simulink model "exLongLinePV_sim"  (R2014b)
settings: Solver=ode45  SolverMode=SingleTasking  StartTime=0.0  StopTime=1.5  MaxStep=0.0015  RelTol=0.0001
values from neighbouring files (symbols this model uses):
  At = full(At)    [exLongLinePV.m]
  Bt = full(Bt)    [exLongLinePV.m]
  bus1_vd = 2^0.5*1e3    (= 1414.21356237)    [ex3busPV.m]    (also in exLongLinePV.m = 141421.356237)
  bus1_vq = 0    [ex3busPV.m]    (also in exLongLinePV.m)
  Cbus = [600e-6 ; 600e-6]    [ex14busSGandPV.m]    (also in exLongLinePV.m = 0.001)
  Cgen = 2e-3*Pren/(gen_vd_init^2+gen_vq_init^2)    (= 5e-07)    [ex3busPV.m]    (also in exLongLinePV.m = 2e-07)
  Ct = full(Ct)    [exLongLinePV.m]
  Dt = full(Dt)    [exLongLinePV.m]
  ki = [0.3 ; 0.3]    [ex14busSGandPV.m]    (also in exLongLinePV.m = 1e-05)
  kp = [1.3e-6 ; 1.3e-6]    [ex14busSGandPV.m]    (also in exLongLinePV.m = 1e-05)
  Pren = [10 ; 10]*1e6    [ex14busSGandPV.m]    (also in ex3busPV.m = 500; exLongLinePV.m = 5000000)
  rel_step = 0.6    [ex3busPV.m]    (also in exLongLinePV.m = 0.02; syncMachVsSwing.m = 1)
  step_time = 9    [ex2busStability.m]    (also in ex3busPV.m = 0.05; exDroopB.m = 10; exLongLinePV.m = 1; syncMachVsSwing.m = 5)
  Vbus_ref = [800 ; 800]    [ex14busSGandPV.m]    (also in exLongLinePV.m = 800)
  ws = 2*pi*50    (= 314.159265359)    [ex14busSGandPV.m]    (also in ex2busStability.m; ex3busPV.m; ex7busLongLine.m; ex9busSG.m)
libraries: simulink x1
settings Model: Creator=COPEC  LastModifiedBy=Juri
settings OptimizationCC: BlockReduction=off  BooleanDataType=off
settings DebuggingCC: SaveWithParameterizedLinksMsg=none  UnderspecifiedInitializationDetection=Classic  MergeDetectMultiDrivingBlocksExec=none  SignalResolutionControl=TryResolveAllWithWarning  SolverPrmCheckMsg=none  FrameProcessingCompatibilityMsg=error
settings HardwareCC: TargetUnknown=on

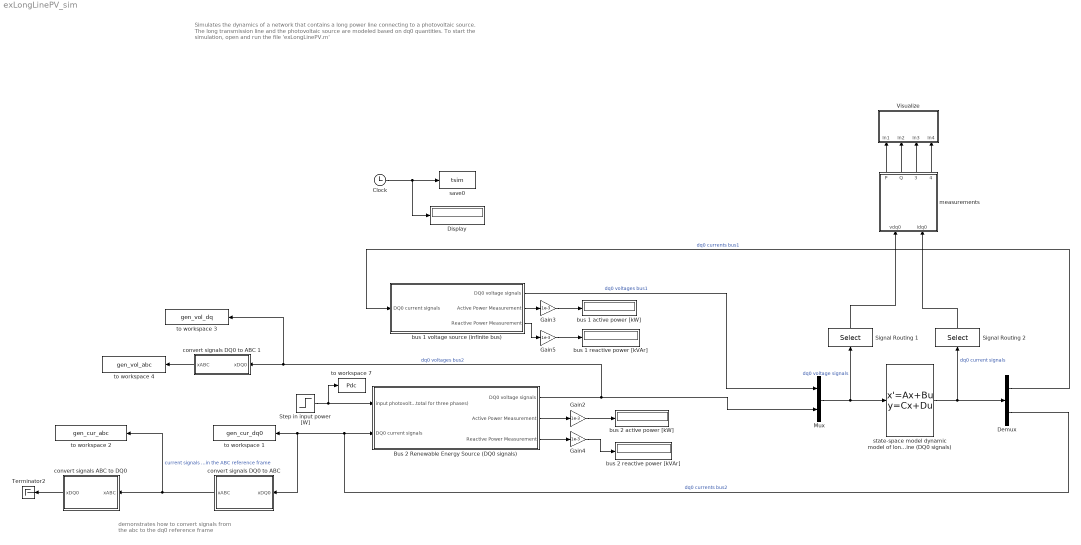
== system exLongLinePV_sim ==
  note: demonstrates how to convert signals
      | from the abc to the dq0 reference frame
  note: Simulates the dynamics of a network that contains
      | a long power line connecting to a photovoltaic source.
      | The long transmission line and the photovoltaic source are modeled
      | based on dq0 quantities.
      |
      | To start the simulation, open and run the file
      | 'exLongLinePV.m'
  Bus 2 Renewable Energy Source (DQ0 signals) : Subsystem
  Clock : Clock
  Demux : Demux  Outputs=2
  Display : Display
  Gain{2..5} (4 alike) : Gain  Gain=1e-3
  Mux : Mux  Inputs=2
  "Signal Routing 1 " : Selector  InputPortWidth=6  IndexOptions=Index vector (dialog)  Indices=[1 4 2 5 3 6]  OutputSizes=1
  Signal Routing 2 : Selector  InputPortWidth=6  IndexOptions=Index vector (dialog)  Indices=[1 4 2 5 3 6]  OutputSizes=1
  Step in input power [W] : Step  Time=step_time  Before=3*Pren  After=3*Pren*(1+rel_step)  SampleTime=0
  Terminator2 : Terminator
  Visualize : Subsystem
  bus 1 voltage source (infinite bus) : Subsystem
  bus 1 active power [kW] : Display
  bus 1 reactive power [kVAr] : Display
  bus 2 active power [kW] : Display
  bus 2 reactive power [kVAr] : Display
  convert signals ABC to DQ0 : Subsystem
  convert signals DQ0 to ABC : Subsystem
  convert signals DQ0 to ABC 1 : Subsystem
  measurements : Subsystem
  save0 : ToWorkspace  VariableName=tsim  SampleTime=-1
  state-space model dynamic model of long transmission line (DQ0 signals) : StateSpace  A=At  B=Bt  C=Ct  D=Dt  X0=0
  to workspace 1 : ToWorkspace  VariableName=gen_cur_dq0  SampleTime=-1
  to workspace 2 : ToWorkspace  VariableName=gen_cur_abc  SampleTime=-1
  to workspace 3 : ToWorkspace  VariableName=gen_vol_dq  SampleTime=-1
  to workspace 4 : ToWorkspace  VariableName=gen_vol_abc  SampleTime=-1
  to workspace 7 : ToWorkspace  VariableName=Pdc  SampleTime=-1
  wires:
  Clock/1 -> Display/1, save0/1
  Gain2/1 -> bus 2 active power [kW]/1
  Gain4/1 -> bus 2 reactive power [kVAr]/1
  Step in input power [W]/1 -> to workspace 7/1, Bus 2 Renewable Energy Source (DQ0 signals)/1(input photovoltaic power (total for three phases))
  Bus 2 Renewable Energy Source (DQ0 signals)/2(Active Power Measurement) -> Gain2/1
  Bus 2 Renewable Energy Source (DQ0 signals)/3("Reactive Power Measurement ") -> Gain4/1
  Mux/1 -> state-space model dynamic model of long transmission line (DQ0 signals)/1, "Signal Routing 1 "/1  "dq0 voltage signals"
  bus 1 voltage source (infinite bus)/1(DQ0 voltage signals) -> Mux/1  "dq0 voltages bus1"
  Bus 2 Renewable Energy Source (DQ0 signals)/1(DQ0 voltage signals) -> to workspace 3/1, convert signals DQ0 to ABC 1/1(xDQ0), Mux/2  "dq0 voltages bus2"
  Demux/1 -> bus 1 voltage source (infinite bus)/1(DQ0 current signals)  "dq0 currents bus1"
  Demux/2 -> Bus 2 Renewable Energy Source (DQ0 signals)/2(DQ0 current signals), convert signals DQ0 to ABC/1(xDQ0), to workspace 1/1  "dq0 currents bus2"
  state-space model dynamic model of long transmission line (DQ0 signals)/1 -> Demux/1, Signal Routing 2/1  "dq0 current signals"
  convert signals DQ0 to ABC/1(xABC) -> to workspace 2/1, convert signals ABC to DQ0/1(xABC)  "current signals in the ABC reference frame"
  convert signals ABC to DQ0/1(xDQ0) -> Terminator2/1
  convert signals DQ0 to ABC 1/1(xABC) -> to workspace 4/1
  bus 1 voltage source (infinite bus)/2(Active Power Measurement) -> Gain3/1
  bus 1 voltage source (infinite bus)/3("Reactive Power Measurement ") -> Gain5/1
  Gain3/1 -> bus 1 active power [kW]/1
  Gain5/1 -> bus 1 reactive power [kVAr]/1
  "Signal Routing 1 "/1 -> measurements/1(vdq0)
  Signal Routing 2/1 -> measurements/2(idq0)
  measurements/1(P) -> Visualize/1(In1)
  measurements/2(Q) -> Visualize/2(In2)
  measurements/3(Vm_RMS) -> Visualize/3(In3)
  measurements/4(Vph_deg) -> Visualize/4(In4)

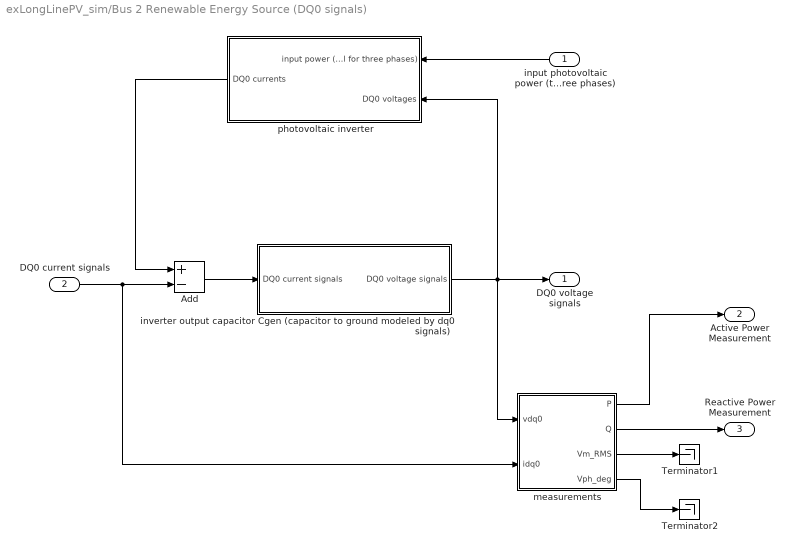
== system exLongLinePV_sim/Bus 2 Renewable Energy Source (DQ0 signals) ==
  input photovoltaic power (total for three phases) : Inport
  DQ0 current signals : Inport  Port=2
  Add : Sum  Inputs=+-
  Terminator1 : Terminator
  Terminator2 : Terminator
  inverter output capacitor Cgen (capacitor to ground modeled by dq0 signals) : Subsystem
  measurements : Subsystem
  photovoltaic inverter : Subsystem
  DQ0 voltage signals : Outport
  Active Power Measurement : Outport  Port=2
  "Reactive Power Measurement " : Outport  Port=3
  wires:
  DQ0 current signals/1 -> Add/2, measurements/2(idq0)
  inverter output capacitor Cgen (capacitor to ground modeled by dq0 signals)/1(DQ0 voltage signals) -> photovoltaic inverter/2(DQ0 voltages), DQ0 voltage signals/1, measurements/1(vdq0)
  input photovoltaic power (total for three phases)/1 -> photovoltaic inverter/1(input power (total for three phases))
  photovoltaic inverter/1(DQ0 currents) -> Add/1
  Add/1 -> inverter output capacitor Cgen (capacitor to ground modeled by dq0 signals)/1(DQ0 current signals)
  measurements/1(P) -> Active Power Measurement/1
  measurements/2(Q) -> "Reactive Power Measurement "/1
  measurements/3(Vm_RMS) -> Terminator1/1
  measurements/4(Vph_deg) -> Terminator2/1

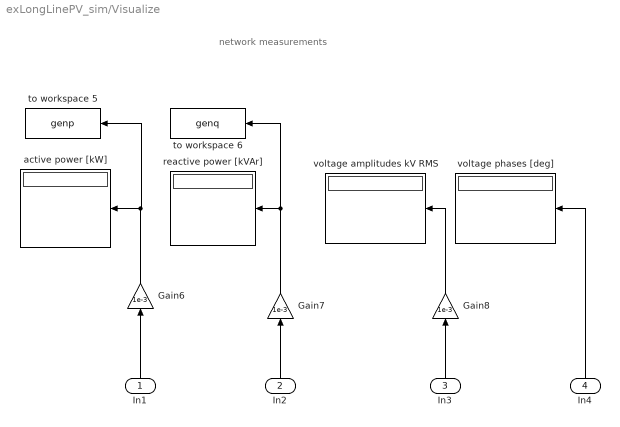
== system exLongLinePV_sim/Visualize ==
  note: network measurements
  In1 : Inport
  In2 : Inport  Port=2
  In3 : Inport  Port=3
  In4 : Inport  Port=4
  Gain6 : Gain  Gain=1e-3
  Gain7 : Gain  Gain=1e-3
  Gain8 : Gain  Gain=1e-3
  active power [kW] : Display
  reactive power [kVAr] : Display
  to workspace 5 : ToWorkspace  VariableName=genp  SampleTime=-1
  to workspace 6 : ToWorkspace  VariableName=genq  SampleTime=-1
  "voltage amplitudes kV RMS " : Display
  voltage phases [deg] : Display
  wires:
  In2/1 -> Gain7/1
  In3/1 -> Gain8/1
  Gain7/1 -> to workspace 6/1, reactive power [kVAr]/1
  In1/1 -> Gain6/1
  Gain8/1 -> "voltage amplitudes kV RMS "/1
  Gain6/1 -> to workspace 5/1, active power [kW]/1
  In4/1 -> voltage phases [deg]/1

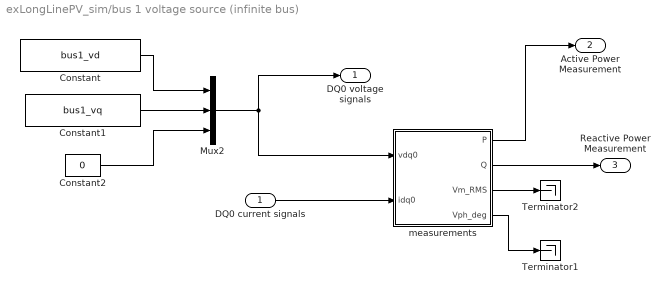
== system exLongLinePV_sim/bus 1 voltage source (infinite bus) ==
  DQ0 current signals : Inport
  Constant : Constant  Value=bus1_vd
  Constant1 : Constant  Value=bus1_vq
  Constant2 : Constant  Value=0
  Mux2 : Mux  Inputs=3
  Terminator1 : Terminator
  Terminator2 : Terminator
  measurements : Subsystem
  DQ0 voltage signals : Outport
  Active Power Measurement : Outport  Port=2
  "Reactive Power Measurement " : Outport  Port=3
  wires:
  Constant/1 -> Mux2/1
  Constant1/1 -> Mux2/2
  Constant2/1 -> Mux2/3
  Mux2/1 -> measurements/1(vdq0), DQ0 voltage signals/1
  DQ0 current signals/1 -> measurements/2(idq0)
  measurements/1(P) -> Active Power Measurement/1
  measurements/2(Q) -> "Reactive Power Measurement "/1
  measurements/3(Vm_RMS) -> Terminator2/1
  measurements/4(Vph_deg) -> Terminator1/1

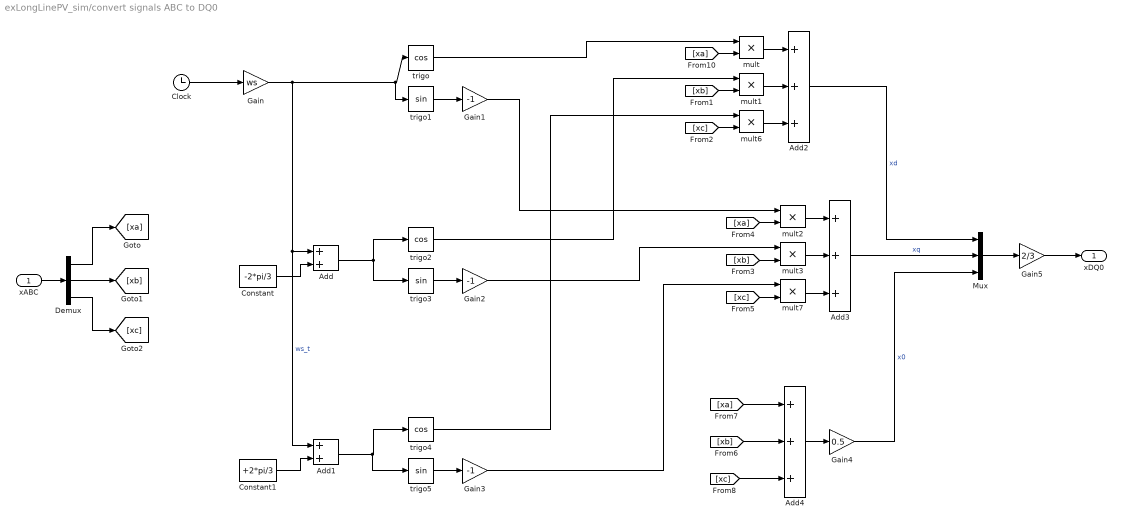
== system exLongLinePV_sim/convert signals ABC to DQ0 ==
  xABC : Inport
  Add : Sum
  Add1 : Sum
  Add2 : Sum  Inputs=+++
  Add3 : Sum  Inputs=+++
  Add4 : Sum  Inputs=+++
  Clock : Clock
  Constant : Constant  Value=-2*pi/3
  Constant1 : Constant  Value=+2*pi/3
  Demux : Demux  Outputs=3
  Gain : Gain  Gain=ws
  Gain1 : Gain  Gain=-1
  Gain2 : Gain  Gain=-1
  Gain3 : Gain  Gain=-1
  Gain4 : Gain  Gain=0.5
  Gain5 : Gain  Gain=2/3
  Mux : Mux  Inputs=3
  mult{,1..3,6..7} (6 alike) : Product  Inputs=**
  trigo : Trigonometry  Operator=cos
  trigo1 : Trigonometry
  trigo2 : Trigonometry  Operator=cos
  trigo3 : Trigonometry
  trigo4 : Trigonometry  Operator=cos
  trigo5 : Trigonometry
  xDQ0 : Outport
  wires:
  Gain5/1 -> xDQ0/1
  Mux/1 -> Gain5/1
  Gain3/1 -> mult7/1
  Gain2/1 -> mult3/1
  Gain1/1 -> mult2/1
  [xc] -> Add4/3
  [xb] -> Add4/2
  [xa] -> Add4/1
  Add4/1 -> Gain4/1
  mult7/1 -> Add3/3
  [xc] -> mult7/2
  [xb] -> mult3/2
  [xa] -> mult2/2
  trigo4/1 -> mult6/1
  mult6/1 -> Add2/3
  [xc] -> mult6/2
  trigo2/1 -> mult1/1
  trigo/1 -> mult/1
  Gain4/1 -> Mux/3  "x0"
  Add3/1 -> Mux/2  "xq"
  Add2/1 -> Mux/1  "xd"
  mult3/1 -> Add3/2
  mult2/1 -> Add3/1
  [xb] -> mult1/2
  [xa] -> mult/2
  mult1/1 -> Add2/2
  mult/1 -> Add2/1
  Demux/3 -> [xc]
  Demux/2 -> [xb]
  Demux/1 -> [xa]
  xABC/1 -> Demux/1
  Add1/1 -> trigo4/1, trigo5/1
  trigo5/1 -> Gain3/1
  Add/1 -> trigo3/1, trigo2/1
  trigo3/1 -> Gain2/1
  trigo1/1 -> Gain1/1
  Constant1/1 -> Add1/2
  Constant/1 -> Add/2
  Gain/1 -> Add/1, Add1/1, trigo/1, trigo1/1  "ws_t"
  Clock/1 -> Gain/1

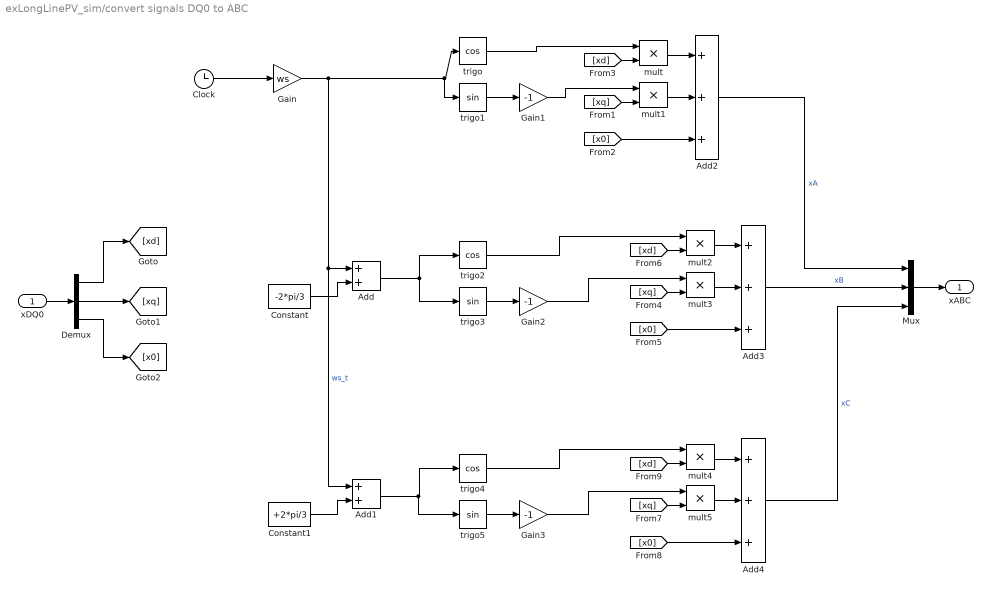
== system exLongLinePV_sim/convert signals DQ0 to ABC ==
  xDQ0 : Inport
  Add : Sum
  Add1 : Sum
  Add2 : Sum  Inputs=+++
  Add3 : Sum  Inputs=+++
  Add4 : Sum  Inputs=+++
  Clock : Clock
  Constant : Constant  Value=-2*pi/3
  Constant1 : Constant  Value=+2*pi/3
  Demux : Demux  Outputs=3
  Gain : Gain  Gain=ws
  Gain1 : Gain  Gain=-1
  Gain2 : Gain  Gain=-1
  Gain3 : Gain  Gain=-1
  Mux : Mux  Inputs=3
  mult{,1..5} (6 alike) : Product  Inputs=**
  trigo : Trigonometry  Operator=cos
  trigo1 : Trigonometry
  trigo2 : Trigonometry  Operator=cos
  trigo3 : Trigonometry
  trigo4 : Trigonometry  Operator=cos
  trigo5 : Trigonometry
  xABC : Outport
  wires:
  Clock/1 -> Gain/1
  Gain/1 -> trigo1/1, trigo/1, Add1/1, Add/1  "ws_t"
  Constant/1 -> Add/2
  Constant1/1 -> Add1/2
  trigo1/1 -> Gain1/1
  trigo3/1 -> Gain2/1
  Add/1 -> trigo2/1, trigo3/1
  trigo5/1 -> Gain3/1
  Add1/1 -> trigo5/1, trigo4/1
  xDQ0/1 -> Demux/1
  Demux/1 -> [xd]
  Demux/2 -> [xq]
  Demux/3 -> [x0]
  Mux/1 -> xABC/1
  mult/1 -> Add2/1
  mult1/1 -> Add2/2
  [xd] -> mult/2
  [xq] -> mult1/2
  [x0] -> Add2/3
  mult2/1 -> Add3/1
  mult3/1 -> Add3/2
  [xd] -> mult2/2
  [xq] -> mult3/2
  [x0] -> Add3/3
  mult4/1 -> Add4/1
  mult5/1 -> Add4/2
  [xd] -> mult4/2
  [xq] -> mult5/2
  [x0] -> Add4/3
  trigo/1 -> mult/1
  Gain1/1 -> mult1/1
  trigo2/1 -> mult2/1
  Gain2/1 -> mult3/1
  trigo4/1 -> mult4/1
  Gain3/1 -> mult5/1
  Add2/1 -> Mux/1  "xA"
  Add3/1 -> Mux/2  "xB"
  Add4/1 -> Mux/3  "xC"

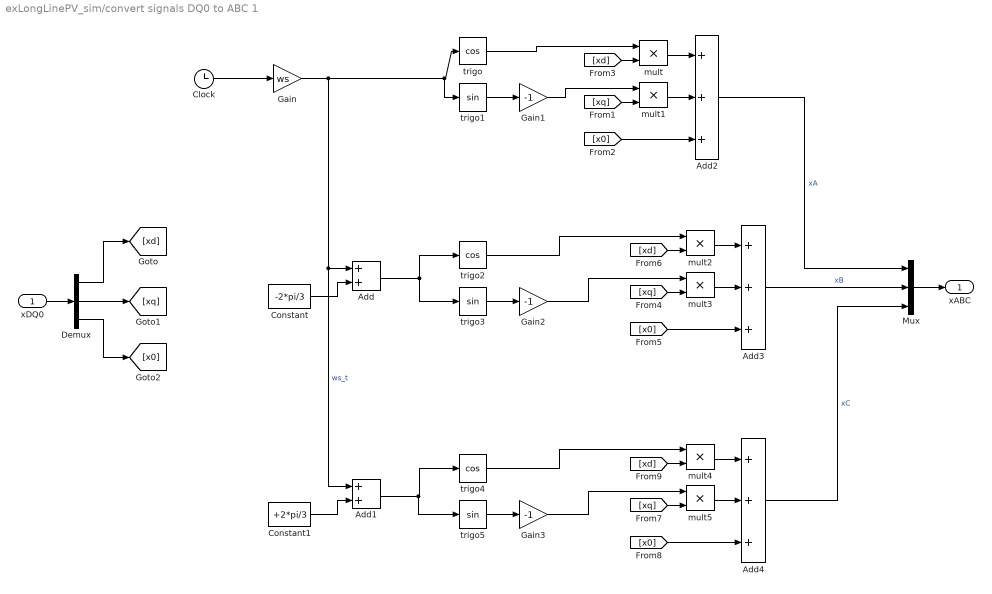
== system exLongLinePV_sim/convert signals DQ0 to ABC 1 ==
  xDQ0 : Inport
  Add : Sum
  Add1 : Sum
  Add2 : Sum  Inputs=+++
  Add3 : Sum  Inputs=+++
  Add4 : Sum  Inputs=+++
  Clock : Clock
  Constant : Constant  Value=-2*pi/3
  Constant1 : Constant  Value=+2*pi/3
  Demux : Demux  Outputs=3
  Gain : Gain  Gain=ws
  Gain1 : Gain  Gain=-1
  Gain2 : Gain  Gain=-1
  Gain3 : Gain  Gain=-1
  Mux : Mux  Inputs=3
  mult{,1..5} (6 alike) : Product  Inputs=**
  trigo : Trigonometry  Operator=cos
  trigo1 : Trigonometry
  trigo2 : Trigonometry  Operator=cos
  trigo3 : Trigonometry
  trigo4 : Trigonometry  Operator=cos
  trigo5 : Trigonometry
  xABC : Outport
  wires:
  Clock/1 -> Gain/1
  Gain/1 -> trigo1/1, trigo/1, Add1/1, Add/1  "ws_t"
  Constant/1 -> Add/2
  Constant1/1 -> Add1/2
  trigo1/1 -> Gain1/1
  trigo3/1 -> Gain2/1
  Add/1 -> trigo2/1, trigo3/1
  trigo5/1 -> Gain3/1
  Add1/1 -> trigo5/1, trigo4/1
  xDQ0/1 -> Demux/1
  Demux/1 -> [xd]
  Demux/2 -> [xq]
  Demux/3 -> [x0]
  Mux/1 -> xABC/1
  mult/1 -> Add2/1
  mult1/1 -> Add2/2
  [xd] -> mult/2
  [xq] -> mult1/2
  [x0] -> Add2/3
  mult2/1 -> Add3/1
  mult3/1 -> Add3/2
  [xd] -> mult2/2
  [xq] -> mult3/2
  [x0] -> Add3/3
  mult4/1 -> Add4/1
  mult5/1 -> Add4/2
  [xd] -> mult4/2
  [xq] -> mult5/2
  [x0] -> Add4/3
  trigo/1 -> mult/1
  Gain1/1 -> mult1/1
  trigo2/1 -> mult2/1
  Gain2/1 -> mult3/1
  trigo4/1 -> mult4/1
  Gain3/1 -> mult5/1
  Add2/1 -> Mux/1  "xA"
  Add3/1 -> Mux/2  "xB"
  Add4/1 -> Mux/3  "xC"

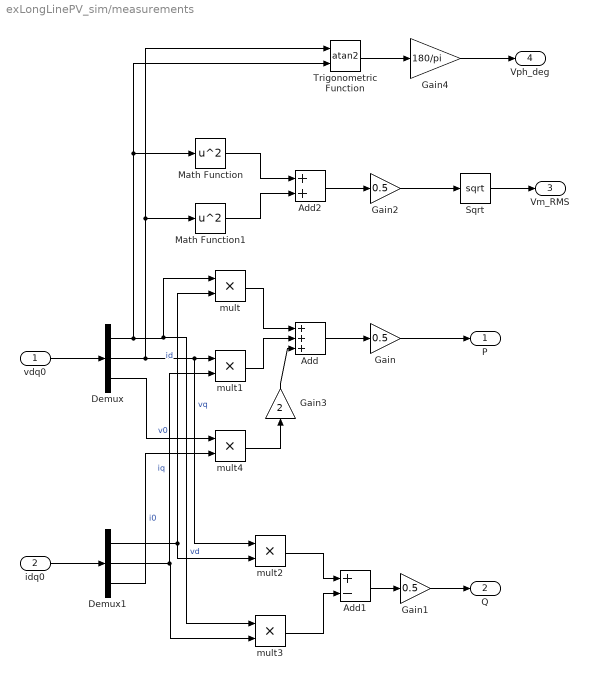
== system exLongLinePV_sim/measurements ==
  vdq0 : Inport
  idq0 : Inport  Port=2
  Add : Sum  Inputs=+++
  Add1 : Sum  Inputs=+-
  Add2 : Sum
  Demux : Demux  Outputs=3
  Demux1 : Demux  Outputs=3
  Gain : Gain  Gain=0.5
  Gain1 : Gain  Gain=0.5
  Gain2 : Gain  Gain=0.5
  Gain3 : Gain  Gain=2
  Gain4 : Gain  Gain=180/pi
  Math Function : Math  Operator=square  SaturateOnIntegerOverflow=on
  Math Function1 : Math  Operator=square  SaturateOnIntegerOverflow=on
  Sqrt : Sqrt  SaturateOnIntegerOverflow=on
  Trigonometric Function : Trigonometry  Operator=atan2
  mult{,1..4} (5 alike) : Product  Inputs=**
  P : Outport
  Q : Outport  Port=2
  Vm_RMS : Outport  Port=3
  Vph_deg : Outport  Port=4
  wires:
  idq0/1 -> Demux1/1
  vdq0/1 -> Demux/1
  Demux/1 -> Math Function/1, Trigonometric Function/2, mult3/1, mult/1  "vd"
  Demux/2 -> Trigonometric Function/1, Math Function1/1, mult2/1, mult1/1  "vq"
  Demux1/1 -> mult/2, mult2/2  "id"
  Demux1/2 -> mult3/2, mult1/2  "iq"
  Demux/3 -> mult4/1  "v0"
  Demux1/3 -> mult4/2  "i0"
  mult/1 -> Add/1
  mult1/1 -> Add/2
  Add/1 -> Gain/1
  mult2/1 -> Add1/1
  mult3/1 -> Add1/2
  Add1/1 -> Gain1/1
  Sqrt/1 -> Vm_RMS/1
  Math Function/1 -> Add2/1
  Math Function1/1 -> Add2/2
  Add2/1 -> Gain2/1
  Gain2/1 -> Sqrt/1
  Gain/1 -> P/1
  Gain1/1 -> Q/1
  mult4/1 -> Gain3/1
  Gain3/1 -> Add/3
  Trigonometric Function/1 -> Gain4/1
  Gain4/1 -> Vph_deg/1

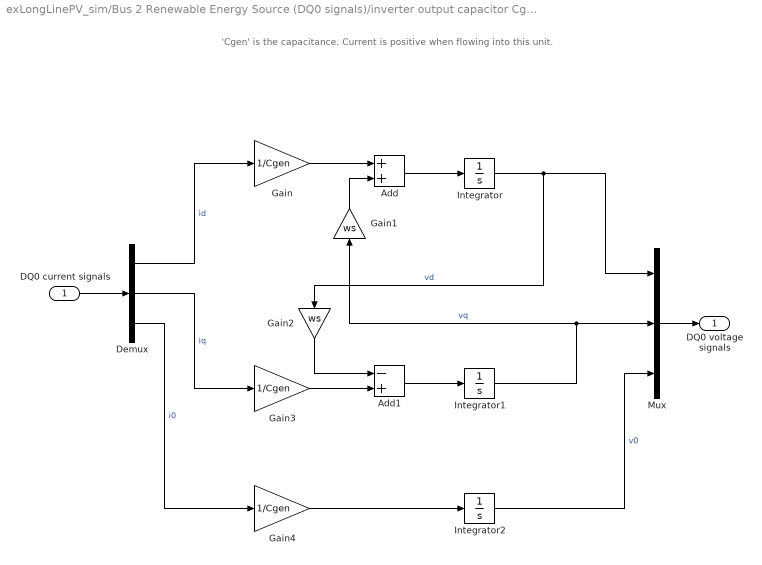
== system exLongLinePV_sim/Bus 2 Renewable Energy Source (DQ0 signals)/inverter output capacitor Cgen (capacitor to ground modeled by dq0 signals) ==
  note: 'Cgen' is the capacitance.
      | Current is positive when flowing into this unit.
  DQ0 current signals : Inport
  Add : Sum
  Add1 : Sum  Inputs=-+
  Demux : Demux  Outputs=3
  Gain : Gain  Gain=1/Cgen
  Gain1 : Gain  Gain=ws
  Gain2 : Gain  Gain=ws
  Gain3 : Gain  Gain=1/Cgen
  Gain4 : Gain  Gain=1/Cgen
  Integrator : Integrator  InitialCondition=bus1_vd
  Integrator1 : Integrator  InitialCondition=bus1_vq
  Integrator2 : Integrator
  Mux : Mux  Inputs=3
  DQ0 voltage signals : Outport
  wires:
  Integrator2/1 -> Mux/3  "v0"
  Mux/1 -> DQ0 voltage signals/1
  Integrator/1 -> Gain2/1, Mux/1  "vd"
  Integrator1/1 -> Gain1/1, Mux/2  "vq"
  Add/1 -> Integrator/1
  Gain1/1 -> Add/2
  DQ0 current signals/1 -> Demux/1
  Demux/1 -> Gain/1  "id"
  Gain/1 -> Add/1
  Add1/1 -> Integrator1/1
  Gain2/1 -> Add1/1
  Demux/2 -> Gain3/1  "iq"
  Gain3/1 -> Add1/2
  Demux/3 -> Gain4/1  "i0"
  Gain4/1 -> Integrator2/1

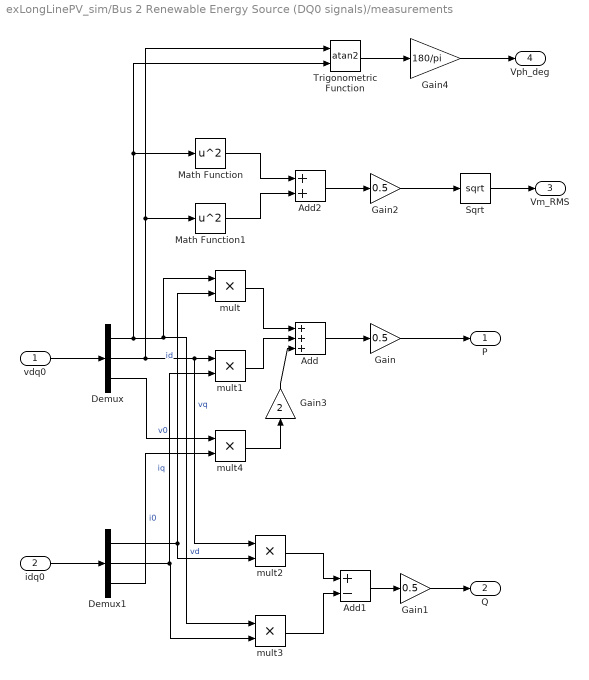
== system exLongLinePV_sim/Bus 2 Renewable Energy Source (DQ0 signals)/measurements ==
  vdq0 : Inport
  idq0 : Inport  Port=2
  Add : Sum  Inputs=+++
  Add1 : Sum  Inputs=+-
  Add2 : Sum
  Demux : Demux  Outputs=3
  Demux1 : Demux  Outputs=3
  Gain : Gain  Gain=0.5
  Gain1 : Gain  Gain=0.5
  Gain2 : Gain  Gain=0.5
  Gain3 : Gain  Gain=2
  Gain4 : Gain  Gain=180/pi
  Math Function : Math  Operator=square  SaturateOnIntegerOverflow=on
  Math Function1 : Math  Operator=square  SaturateOnIntegerOverflow=on
  Sqrt : Sqrt  SaturateOnIntegerOverflow=on
  Trigonometric Function : Trigonometry  Operator=atan2
  mult{,1..4} (5 alike) : Product  Inputs=**
  P : Outport
  Q : Outport  Port=2
  Vm_RMS : Outport  Port=3
  Vph_deg : Outport  Port=4
  wires:
  idq0/1 -> Demux1/1
  vdq0/1 -> Demux/1
  Demux/1 -> Math Function/1, Trigonometric Function/2, mult3/1, mult/1  "vd"
  Demux/2 -> Trigonometric Function/1, Math Function1/1, mult2/1, mult1/1  "vq"
  Demux1/1 -> mult/2, mult2/2  "id"
  Demux1/2 -> mult3/2, mult1/2  "iq"
  Demux/3 -> mult4/1  "v0"
  Demux1/3 -> mult4/2  "i0"
  mult/1 -> Add/1
  mult1/1 -> Add/2
  Add/1 -> Gain/1
  mult2/1 -> Add1/1
  mult3/1 -> Add1/2
  Add1/1 -> Gain1/1
  Sqrt/1 -> Vm_RMS/1
  Math Function/1 -> Add2/1
  Math Function1/1 -> Add2/2
  Add2/1 -> Gain2/1
  Gain2/1 -> Sqrt/1
  Gain/1 -> P/1
  Gain1/1 -> Q/1
  mult4/1 -> Gain3/1
  Gain3/1 -> Add/3
  Trigonometric Function/1 -> Gain4/1
  Gain4/1 -> Vph_deg/1

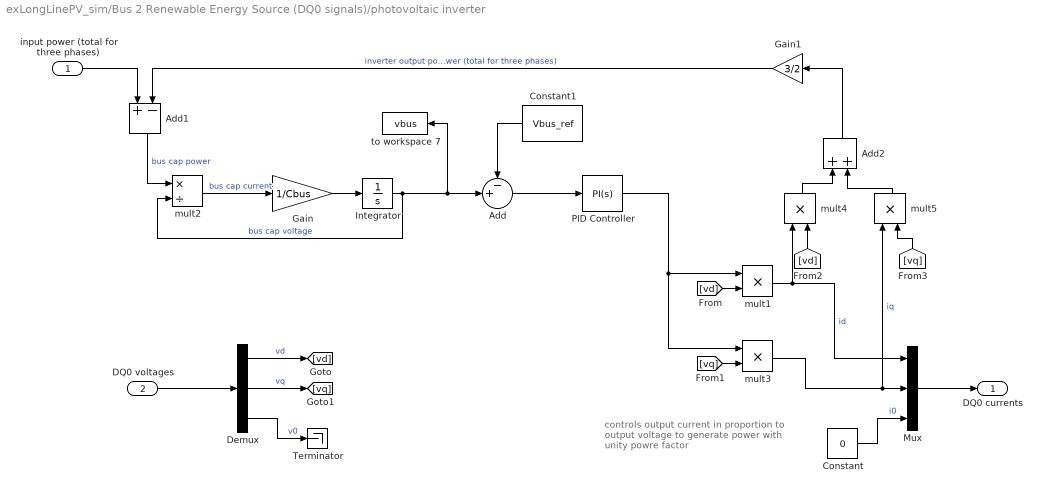
== system exLongLinePV_sim/Bus 2 Renewable Energy Source (DQ0 signals)/photovoltaic inverter ==
  note: controls output current in proportion
      | to output voltage to generate power
      | with unity powre factor
  input power (total for three phases) : Inport
  DQ0 voltages : Inport  Port=2
  Add : Sum  Inputs=-+|
  Add1 : Sum  Inputs=+-
  Add2 : Sum
  Constant : Constant  Value=0
  Constant1 : Constant  Value=Vbus_ref
  Demux : Demux  Outputs=3
  Gain : Gain  Gain=1/Cbus
  Gain1 : Gain  Gain=3/2
  Integrator : Integrator  InitialCondition=Vbus_ref*0.8
  Mux : Mux  Inputs=3
  PID Controller : simulink/Continuous/PID Controller  Controller=PI  TimeDomain=Continuous-time  SampleTime=-1  IntegratorMethod=Forward Euler  FilterMethod=Forward Euler  Form=Parallel  UseFilter=on  ControllerParametersSource=internal  P=kp  I=ki  D=0  N=100  InitialConditionSource=internal  InitialConditionForIntegrator=0  InitialConditionForFilter=0  ExternalReset=none  LimitOutput=off  UpperSaturationLimit=inf  LowerSaturationLimit=-inf  LinearizeAsGain=on  AntiWindupMode=none  Kb=1  TrackingMode=off  Kt=1  PParamMin=[]  PParamMax=[]  IParamMin=[]  IParamMax=[]  DParamMin=[]  DParamMax=[]  NParamMin=[]  NParamMax=[]  KbParamMin=[]  KbParamMax=[]  KtParamMin=[]  KtParamMax=[]  POutMin=[]  POutMax=[]  IOutMin=[]  IOutMax=[]  DOutMin=[]  DOutMax=[]  NOutMin=[]  NOutMax=[]  KbOutMin=[]  KbOutMax=[]  KtOutMin=[]  KtOutMax=[]  IntegratorOutMin=[]  IntegratorOutMax=[]  FilterOutMin=[]  FilterOutMax=[]  SumOutMin=[]  SumOutMax=[]  SumI1OutMin=[]  SumI1OutMax=[]  SumI2OutMin=[]  SumI2OutMax=[]  SumI3OutMin=[]  SumI3OutMax=[]  SumDOutMin=[]  SumDOutMax=[]  SaturationOutMin=[]  SaturationOutMax=[]  IntegratorContinuousStateAttributes=''  IntegratorStateMustResolveToSignalObject=off  IntegratorRTWStateStorageClass=Auto  FilterContinuousStateAttributes=''  FilterStateMustResolveToSignalObject=off  FilterRTWStateStorageClass=Auto  DifferentiatorICPrevScaledInput=0  DifferentiatorOutMin=[]  DifferentiatorOutMax=[]
  Terminator : Terminator
  mult{1,3..5} (4 alike) : Product  Inputs=**
  mult2 : Product  Inputs=*/
  to workspace 7 : ToWorkspace  VariableName=vbus  SampleTime=-1
  DQ0 currents : Outport
  wires:
  DQ0 voltages/1 -> Demux/1
  Demux/3 -> Terminator/1  "v0"
  Mux/1 -> DQ0 currents/1
  mult1/1 -> mult4/1, Mux/1  "id"
  mult3/1 -> mult5/1, Mux/2  "iq"
  Constant/1 -> Mux/3  "i0"
  Demux/1 -> [vd]  "vd"
  Demux/2 -> [vq]  "vq"
  PID Controller/1 -> mult1/1, mult3/1
  Add/1 -> PID Controller/1
  Constant1/1 -> Add/1
  Integrator/1 -> mult2/2, to workspace 7/1, Add/2  "bus cap voltage"
  mult2/1 -> Gain/1  "bus cap current"
  Gain/1 -> Integrator/1
  Add1/1 -> mult2/1  "bus cap power"
  input power (total for three phases)/1 -> Add1/1
  Gain1/1 -> Add1/2  "inverter output power (total for three phases)"
  [vd] -> mult1/2
  [vq] -> mult3/2
  [vd] -> mult4/2
  [vq] -> mult5/2
  mult4/1 -> Add2/1
  mult5/1 -> Add2/2
  Add2/1 -> Gain1/1

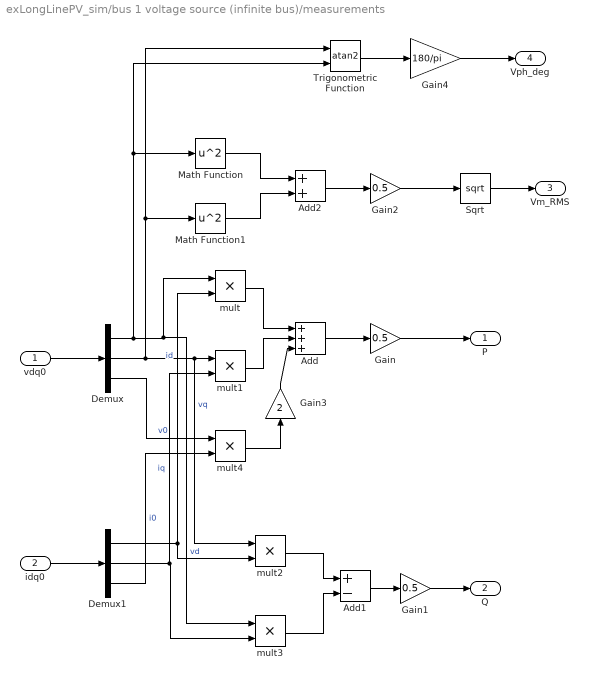
== system exLongLinePV_sim/bus 1 voltage source (infinite bus)/measurements ==
  vdq0 : Inport
  idq0 : Inport  Port=2
  Add : Sum  Inputs=+++
  Add1 : Sum  Inputs=+-
  Add2 : Sum
  Demux : Demux  Outputs=3
  Demux1 : Demux  Outputs=3
  Gain : Gain  Gain=0.5
  Gain1 : Gain  Gain=0.5
  Gain2 : Gain  Gain=0.5
  Gain3 : Gain  Gain=2
  Gain4 : Gain  Gain=180/pi
  Math Function : Math  Operator=square  SaturateOnIntegerOverflow=on
  Math Function1 : Math  Operator=square  SaturateOnIntegerOverflow=on
  Sqrt : Sqrt  SaturateOnIntegerOverflow=on
  Trigonometric Function : Trigonometry  Operator=atan2
  mult{,1..4} (5 alike) : Product  Inputs=**
  P : Outport
  Q : Outport  Port=2
  Vm_RMS : Outport  Port=3
  Vph_deg : Outport  Port=4
  wires:
  idq0/1 -> Demux1/1
  vdq0/1 -> Demux/1
  Demux/1 -> Math Function/1, Trigonometric Function/2, mult3/1, mult/1  "vd"
  Demux/2 -> Trigonometric Function/1, Math Function1/1, mult2/1, mult1/1  "vq"
  Demux1/1 -> mult/2, mult2/2  "id"
  Demux1/2 -> mult3/2, mult1/2  "iq"
  Demux/3 -> mult4/1  "v0"
  Demux1/3 -> mult4/2  "i0"
  mult/1 -> Add/1
  mult1/1 -> Add/2
  Add/1 -> Gain/1
  mult2/1 -> Add1/1
  mult3/1 -> Add1/2
  Add1/1 -> Gain1/1
  Sqrt/1 -> Vm_RMS/1
  Math Function/1 -> Add2/1
  Math Function1/1 -> Add2/2
  Add2/1 -> Gain2/1
  Gain2/1 -> Sqrt/1
  Gain/1 -> P/1
  Gain1/1 -> Q/1
  mult4/1 -> Gain3/1
  Gain3/1 -> Add/3
  Trigonometric Function/1 -> Gain4/1
  Gain4/1 -> Vph_deg/1
